simulink model "helicopter4_yes_flys_manually_and_auto"  (Simulink 8.0)
settings: Solver=ode45  StartTime=0.0  StopTime=inf  RelTol=1e-3
libraries: etargetslib x2, dspnetwork x2, simulink x1, vrlib x1, aerolibanimutils x1
settings Model: Creator=cheki_000  LastModifiedBy=Администратор
settings DebuggingCC: MultiTaskDSMMsg=warning  MultiTaskCondExecSysMsg=none  FcnCallInpInsideContextMsg=EnableAllAsWarning  StrictBusMsg=None
settings RTWCC: IncludeERTFirstTime=on

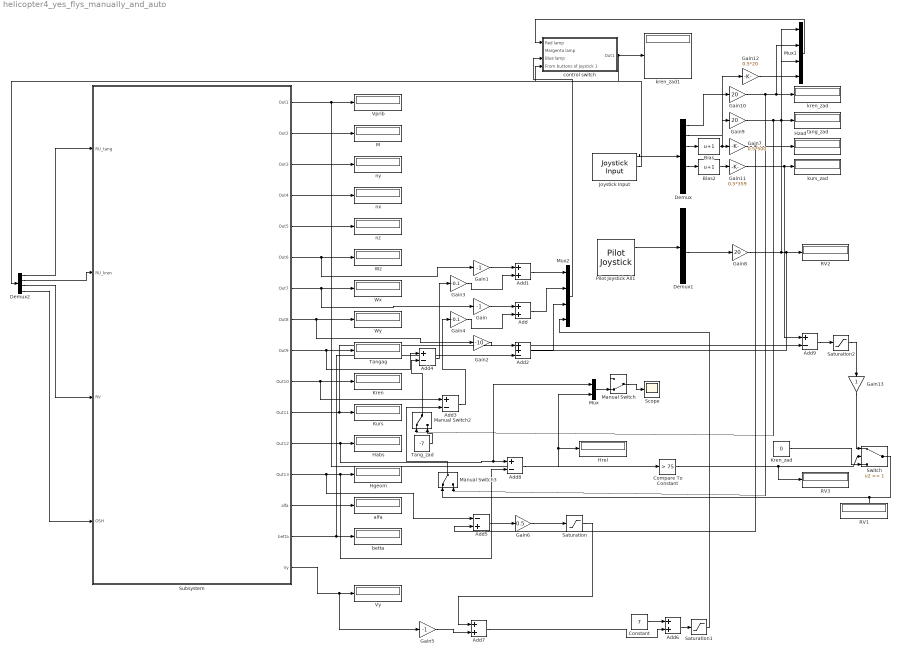
== system helicopter4_yes_flys_manually_and_auto ==
  Add{,1,6..7} (4 alike) : Sum
  Add2 : Sum  Inputs=++-
  Add{3..4,8..9} (4 alike) : Sum  Inputs=+-
  Add5 : Sum  Inputs=-+
  Bias : Bias  Bias=1
  Bias2 : Bias  Bias=1
  Compare To Constant : simulink/Logic and Bit Operations/Compare To Constant  relop=>  const=75  OutDataTypeStr=uint8
  Constant : Constant  Value=7
  Demux : Demux  Outputs=7
  Demux1 : Demux  Outputs=6
  Demux2 : Demux
  Gain : Gain  Gain=-1
  Gain1 : Gain  Gain=-1
  Gain10 : Gain  Gain=20
  Gain11 : Gain  Gain=0.5*359
  Gain12 : Gain  Gain=0.5*20
  Gain13 : Gain
  Gain2 : Gain  Gain=-10
  Gain3 : Gain  Gain=-0.1
  Gain4 : Gain  Gain=-0.1
  Gain5 : Gain  Gain=-1
  Gain6 : Gain  Gain=0.5
  Gain7 : Gain  Gain=0.5*500
  Gain8 : Gain  Gain=20
  Gain9 : Gain  Gain=20
  Habs : Display
  Hgeom : Display
  Hrel : Display
  Joystick Input : vrlib/Joystick Input  joyid=1  adjustports=on  forcefeed=off
  Kren : Display
  Kren_zad : Constant  Value=0
  Kurs : Display
  M : Display
  Manual Switch : ManualSwitch  CurrentSetting=0
  Manual Switch2 : ManualSwitch
  Manual Switch3 : ManualSwitch
  Mux : Mux  Inputs=2
  Mux1 : Mux
  Mux2 : Mux
  Pilot Joystick All1 : aerolibanimutils/Pilot Joystick  JoystickID=Joystick2  OutputConfiguration=AllOutputs  SampleTime=1/30
  RV1 : Display
  RV2 : Display
  RV3 : Display
  Saturation : Saturate  UpperLimit=10  LowerLimit=-10
  Saturation1 : Saturate  UpperLimit=18  LowerLimit=0
  Saturation2 : Saturate  UpperLimit=30  LowerLimit=-30
  Scope : Scope
      settings: TimeRange=1200  YMin=850  YMax=1175  MaxDataPoints=500000
  Subsystem : Subsystem
  Switch : Switch  Threshold=1
  Tang_zad : Constant  Value=-7
  Tangag : Display
  Vprib : Display
  Vy : Display
  Wx : Display
  Wy : Display
  Wz : Display
  alfa : Display
  betta : Display
  control switch : Subsystem
  kren_zad : Display
  kren_zad1 : Display
  kurs_zad : Display
  nx : Display
  ny : Display
  nz : Display
  tang_zad : Display
  Нzad : Display
  wires:
  Subsystem/10(Out10) -> Add3/1, Kren/1
  Subsystem/11(Out11) -> Kurs/1, Add9/2
  Subsystem/13(Out13) -> Add5/1, Add8/2, Hgeom/1
  Subsystem/12(Out12) -> Mux/1, Add8/1, Habs/1
  Subsystem/6(Out6) -> Gain1/1, Wz/1
  Subsystem/7(Out7) -> Gain/1, Wx/1
  Subsystem/8(Out8) -> Gain2/1, Wy/1
  Subsystem/2(Out2) -> M/1
  Subsystem/5(Out5) -> nz/1
  Subsystem/4(Out4) -> nx/1
  Subsystem/3(Out3) -> ny/1
  Subsystem/1(Out1) -> Vprib/1, Compare To Constant/1
  Subsystem/9(Out9) -> Add4/1, Tangag/1
  Subsystem/14(alfa) -> alfa/1
  Subsystem/15(betta) -> betta/1, Add2/3
  Gain/1 -> Add/1
  Gain1/1 -> Add1/1
  Gain2/1 -> Add2/1
  Gain3/1 -> Add1/2
  Gain4/1 -> Add/2
  Add3/1 -> Gain4/1
  Add4/1 -> Gain3/1
  Subsystem/16(Vy) -> Gain5/1, Vy/1
  Constant/1 -> Add6/1
  Gain5/1 -> Add7/2
  Add5/1 -> Gain6/1
  Gain6/1 -> Saturation/1
  Saturation/1 -> Add7/1
  Add8/1 -> Mux/2, Hrel/1
  Mux/1 -> Manual Switch/2
  Manual Switch/1 -> Scope/1
  Joystick Input/1 -> Demux/1
  Pilot Joystick All1/1 -> Demux1/1
  Gain7/1 -> Нzad/1, Add5/2
  Demux/3 -> Bias/1
  Bias/1 -> Gain7/1, Gain12/1
  Demux1/4 -> Gain8/1
  Gain8/1 -> Mux1/3, RV2/1, Add2/2
  Demux/2 -> Gain9/1
  Gain9/1 -> Manual Switch2/1, tang_zad/1, Mux1/1
  Tang_zad/1 -> Manual Switch2/2
  Manual Switch2/1 -> Add4/2
  Demux/1 -> Gain10/1
  Gain10/1 -> kren_zad/1, Mux1/2, Manual Switch3/2
  Demux/5 -> Bias2/1
  Bias2/1 -> Gain11/1
  Gain11/1 -> kurs_zad/1, Add9/1
  Manual Switch3/1 -> Add3/2
  Gain12/1 -> Mux1/4
  Mux1/1 -> control switch/1(Red lamp)
  control switch/1(Out1) -> Demux2/1, kren_zad1/1
  Joystick Input/2 -> control switch/4(From buttons of joystick 1)
  Add1/1 -> Mux2/1
  Add/1 -> Mux2/2
  Add2/1 -> Mux2/3
  Add6/1 -> Saturation1/1
  Add7/1 -> Add6/2
  Saturation1/1 -> Mux2/4
  Mux2/1 -> control switch/3(Blue lamp)
  Demux2/1 -> Subsystem/1(RU_tang)
  Demux2/2 -> Subsystem/2(RU_kren)
  Demux2/3 -> Subsystem/3(RV)
  Demux2/4 -> Subsystem/4(OSH)
  Compare To Constant/1 -> Switch/2, RV3/1
  Add9/1 -> Saturation2/1
  Saturation2/1 -> Gain13/1
  Switch/1 -> Manual Switch3/1, RV1/1
  Gain13/1 -> Switch/1
  Kren_zad/1 -> Switch/3

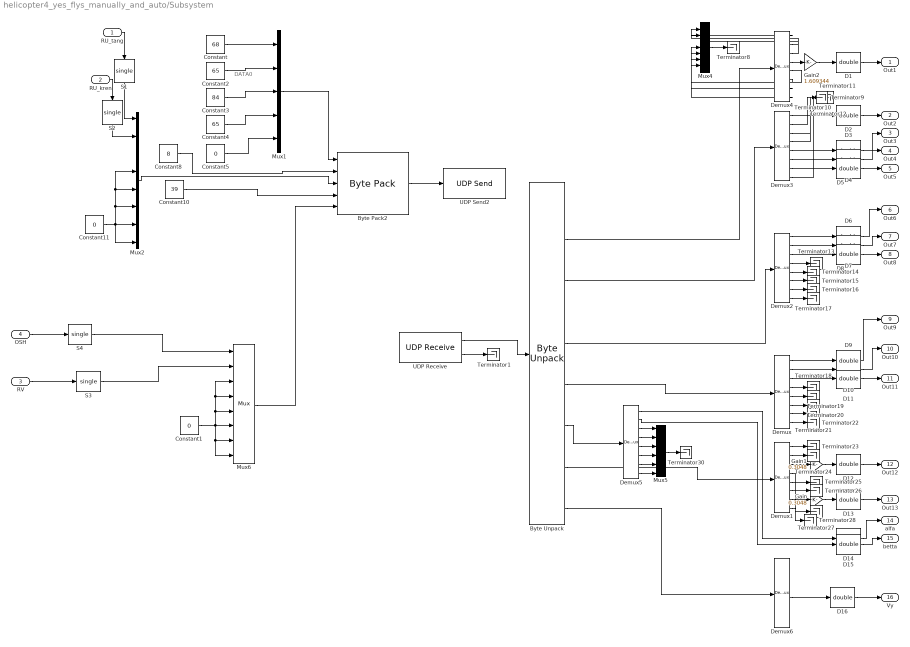
== system helicopter4_yes_flys_manually_and_auto/Subsystem ==
  note: DATA0
  RU_tang : Inport
  RU_kren : Inport  Port=2
  RV : Inport  Port=3
  OSH : Inport  Port=4
  Byte Pack2 : etargetslib/Byte Pack  datatypes={'int8','int32','single','int32','single'}  byteAlign=1
  Byte Unpack : etargetslib/Byte Unpack  dimensions={[5+3*36],[1],[8],[1],[8],[12*36],[1],[8],[1],[8],[1],[8],[1],[8],[1],[8]}  datatypes={'int8','int32','single','int32','single','int8','int32','single','int32','single','int32','single','int32','single','int32','single'}  byteAlign=1
  Constant : Constant  Value=68  OutDataTypeStr=int8
  Constant1 : Constant  Value=0  OutDataTypeStr=single  LockScale=on
  Constant10 : Constant  Value=39  OutDataTypeStr=int32  LockScale=on
  Constant11 : Constant  Value=0  OutDataTypeStr=single  LockScale=on
  Constant2 : Constant  Value=65  OutDataTypeStr=int8  LockScale=on
  Constant3 : Constant  Value=84  OutDataTypeStr=int8
  Constant4 : Constant  Value=65  OutDataTypeStr=int8  LockScale=on
  Constant5 : Constant  Value=0  OutDataTypeStr=int8  LockScale=on
  Constant8 : Constant  Value=8  OutDataTypeStr=int32  LockScale=on
  D{1..16} (16 alike) : DataTypeConversion  OutDataTypeStr=double
  Demux{,1..6} (7 alike) : Demux  Outputs=8
  Gain : Gain  Gain=0.3048
  Gain1 : Gain  Gain=0.3048
  Gain2 : Gain  Gain=1.609344
  Mux1 : Mux  Inputs=5
  Mux2 : Mux  Inputs=8
  Mux4 : Mux  Inputs=7
  Mux5 : Mux  Inputs=6
  Mux6 : Mux  Inputs=8
  S{1..4} (4 alike) : DataTypeConversion  OutDataTypeStr=single
  Terminator{1,8..28,30} (23 alike) : Terminator
  UDP Receive : dspnetwork/UDP Receive  localURL='0.0.0.0'  localPort=4444  remoteURL='192.168.1.1'  remotePort=-1  recvBufferSize=8192  dims=720+5+36+36  signalDatatype=uint8  isVarSize=off  showBlockingTime=off  blockingTime=0  sampletime=inf
  UDP Send2 : dspnetwork/UDP Send  remoteURL='192.168.1.1'  remotePort=49000  localURL='0.0.0.0'  localPortSource=Automatically determine  localPort=4444  sampletime=-1  separateLengthPort=0
  Out1 : Outport
  Out2 : Outport  Port=2
  Out3 : Outport  Port=3
  Out4 : Outport  Port=4
  Out5 : Outport  Port=5
  Out6 : Outport  Port=6
  Out7 : Outport  Port=7
  Out8 : Outport  Port=8
  Out9 : Outport  Port=9
  Out10 : Outport  Port=10
  Out11 : Outport  Port=11
  Out12 : Outport  Port=12
  Out13 : Outport  Port=13
  alfa : Outport  Port=14
  betta : Outport  Port=15
  Vy : Outport  Port=16
  wires:
  Constant/1 -> Mux1/1
  Constant2/1 -> Mux1/2
  Constant3/1 -> Mux1/3
  Constant4/1 -> Mux1/4
  Constant5/1 -> Mux1/5
  Mux1/1 -> Byte Pack2/1
  Byte Pack2/1 -> UDP Send2/1
  Constant8/1 -> Byte Pack2/2
  Mux2/1 -> Byte Pack2/3
  Demux1/4 -> Gain/1
  Demux1/3 -> Gain1/1
  Byte Unpack/8 -> Demux2/1
  Byte Unpack/5 -> Demux3/1
  Demux4/4 -> Gain2/1
  Byte Unpack/3 -> Demux4/1
  OSH/1 -> S4/1
  Demux4/1 -> Mux4/1
  Demux4/2 -> Mux4/2
  Demux4/3 -> Mux4/3
  Demux4/5 -> Mux4/4
  Demux4/6 -> Mux4/5
  Demux4/7 -> Mux4/6
  Demux4/8 -> Mux4/7
  Mux4/1 -> Terminator8/1
  Demux3/2 -> Terminator9/1
  Demux3/3 -> Terminator10/1
  Demux3/4 -> Terminator11/1
  Demux3/8 -> Terminator12/1
  Demux2/4 -> Terminator13/1
  Demux2/5 -> Terminator14/1
  Demux2/6 -> Terminator15/1
  Demux2/7 -> Terminator16/1
  Demux2/8 -> Terminator17/1
  Demux/4 -> Terminator18/1
  Demux/5 -> Terminator19/1
  Demux/6 -> Terminator20/1
  Demux/7 -> Terminator21/1
  Demux/8 -> Terminator22/1
  Demux1/1 -> Terminator23/1
  Demux1/2 -> Terminator24/1
  Demux1/5 -> Terminator25/1
  Demux1/6 -> Terminator26/1
  Demux1/7 -> Terminator27/1
  Demux1/8 -> Terminator28/1
  Constant11/1 -> Mux2/7, Mux2/4, Mux2/5, Mux2/6, Mux2/8
  Gain2/1 -> D1/1
  Demux3/1 -> D2/1
  RU_tang/1 -> S1/1
  RU_kren/1 -> S2/1
  Demux3/5 -> D3/1
  RV/1 -> S3/1
  Demux3/6 -> D4/1
  Demux3/7 -> D5/1
  Demux2/1 -> D6/1
  Demux2/2 -> D7/1
  Demux2/3 -> D8/1
  Demux/1 -> D9/1
  Demux/2 -> D10/1
  Demux/3 -> D11/1
  Gain1/1 -> D12/1
  Gain/1 -> D13/1
  D1/1 -> Out1/1
  D2/1 -> Out2/1
  D3/1 -> Out3/1
  D4/1 -> Out4/1
  D5/1 -> Out5/1
  D6/1 -> Out6/1
  D7/1 -> Out7/1
  D8/1 -> Out8/1
  D9/1 -> Out9/1
  D10/1 -> Out10/1
  D11/1 -> Out11/1
  D12/1 -> Out12/1
  D13/1 -> Out13/1
  S1/1 -> Mux2/1
  S2/1 -> Mux2/2
  S4/1 -> Mux6/1
  Byte Unpack/12 -> Demux5/1
  Demux5/1 -> D14/1
  Demux5/2 -> D15/1
  Demux5/3 -> Mux5/1
  Demux5/4 -> Mux5/2
  Demux5/5 -> Mux5/3
  Demux5/6 -> Mux5/4
  Demux5/7 -> Mux5/5
  Demux5/8 -> Mux5/6
  Mux5/1 -> Terminator30/1
  D14/1 -> alfa/1
  D15/1 -> betta/1
  Constant10/1 -> Byte Pack2/4
  UDP Receive/1 -> Byte Unpack/1
  Byte Unpack/10 -> Demux/1
  Constant1/1 -> Mux6/8, Mux6/7, Mux6/3, Mux6/4, Mux6/5, Mux6/6
  Mux6/1 -> Byte Pack2/5
  S3/1 -> Mux6/2
  Byte Unpack/14 -> Demux1/1
  UDP Receive/2 -> Terminator1/1
  Byte Unpack/16 -> Demux6/1
  Demux6/5 -> D16/1
  D16/1 -> Vy/1

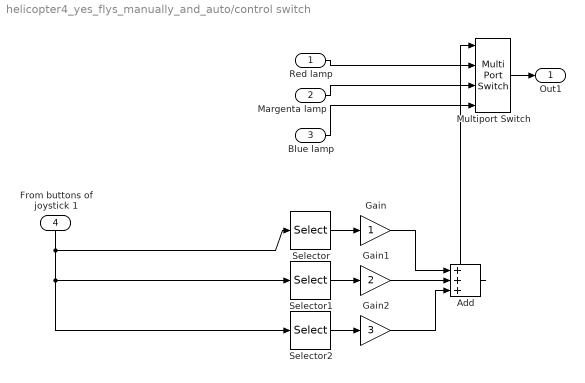
== system helicopter4_yes_flys_manually_and_auto/control switch ==
  Red lamp : Inport
  Margenta lamp : Inport  Port=2
  Blue lamp : Inport  Port=3
  From buttons of joystick 1 : Inport  Port=4
  Add : Sum  Inputs=+++
  Gain : Gain
  Gain1 : Gain  Gain=2
  Gain2 : Gain  Gain=3
  Multiport Switch : MultiPortSwitch  DiagnosticForDefault=None
  Selector : Selector  InputPortWidth=39  IndexOptions=Index vector (dialog)  Indices=[28]  OutputSizes=1
  Selector1 : Selector  InputPortWidth=39  IndexOptions=Index vector (dialog)  Indices=[29]  OutputSizes=1
  Selector2 : Selector  InputPortWidth=39  IndexOptions=Index vector (dialog)  Indices=[30]  OutputSizes=1
  Out1 : Outport
  wires:
  Selector/1 -> Gain/1
  Selector1/1 -> Gain1/1
  Gain1/1 -> Add/2
  Selector2/1 -> Gain2/1
  Gain2/1 -> Add/3
  Gain/1 -> Add/1
  Add/1 -> Multiport Switch/1
  From buttons of joystick 1/1 -> Selector1/1, Selector2/1, Selector/1
  Red lamp/1 -> Multiport Switch/2
  Multiport Switch/1 -> Out1/1
  Margenta lamp/1 -> Multiport Switch/3
  Blue lamp/1 -> Multiport Switch/4
